simulink model "model"  (R2017b)
settings: Solver=VariableStepAuto  StartTime=0.0  StopTime=10.0  RelTol=1e-3  EnableMultiTasking=on
values from neighbouring files (symbols this model uses):
  A = zeros(5,5)    [kalmanfilter.m]    (also in model_2017.m = [[0  0   0   0                0             0   1           ; model_rough.m; model_v2.m = [[0  0   0   0                0             0   1           ; model_v3.m = [[0  0   0   0                0             0   1           )
  B = zeros(5,6)    [kalmanfilter.m]    (also in model_2017.m = [[0      0      0      0     ];                        [0   ; model_rough.m; model_v2.m = [[0      0      0      0     ];                        [0   ; model_v3.m = [[0      0      0      0      0      0             ];       )
  C = eye(5)    [kalmanfilter.m]    (also in model_2017.m = [[0  0   0   0   0   0   1   0   0   0   0   0]; model_rough.m; model_v2.m = [[0  0   0   0   0   0   1   0   0   0   0   0]; model_v3.m = [[0  0   0   0   0   0   1   0   0   0   0   0])
settings Model: Creator=nagamune  LastModifiedBy=Carter
settings DataIOCC: LimitDataPoints=on  SaveFormat=Array
settings OptimizationCC: LifeSpan=inf
settings DebuggingCC: SolverPrmCheckMsg=warning  SFUnexpectedBacktrackingDiag=warning  SFNoUnconditionalDefaultTransitionDiag=warning  SFExecutionAtInitializationDiag=none
settings HardwareCC: ProdBitPerPointer=32  ProdBitPerSizeT=32  ProdBitPerPtrDiffT=32  ProdLargestAtomicFloat=None  ProdIntDivRoundTo=Undefined  ProdEndianess=Unspecified  ProdWordSize=32  ProdHWDeviceType=32-bit Generic
settings ModelReferenceCC: PropagateSignalLabelsOutOfModel=off
settings CodeAppCC: StateflowObjectComments=on
settings GRTTargetCC: TargetLangStandard=C89/C90 (ANSI)  GeneratePreprocessorConditionals=Disable all
settings ConfigComp: CovMetricSettings=dw  CovHtmlReporting=on  CovSaveCumulativeToWorkspaceVar=on  CovSaveSingleToWorkspaceVar=on  CovExternalEMLEnable=off  CovSFcnEnable=off

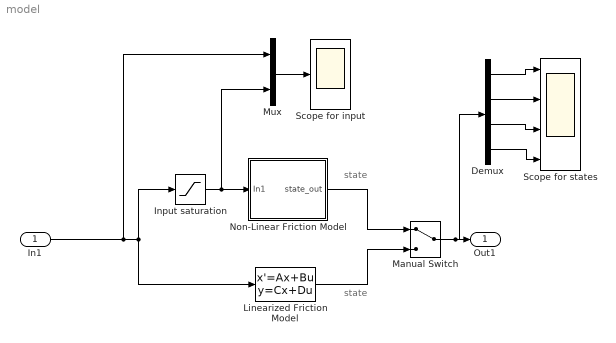
== system model ==
  note: state
  note: state
  In1 : Inport
  Demux : Demux
  Input saturation : Saturate  UpperLimit=10  LowerLimit=-10
  Linearized Friction Model : StateSpace  A=A  B=B  C=C  D=zeros(5,6)  InitialCondition=[0.3 0 0 0 0]
  Manual Switch : ManualSwitch
  Mux : Mux  Inputs=2
  Non-Linear Friction Model : Subsystem
  Scope for input : Scope
  Scope for states : Scope  NumInputPorts=4
  Out1 : Outport
  wires:
  Non-Linear Friction Model/1(state_out) -> Manual Switch/1
  Linearized Friction Model/1 -> Manual Switch/2
  In1/1 -> Mux/1, Linearized Friction Model/1, Input saturation/1
  Manual Switch/1 -> Demux/1, Out1/1
  Input saturation/1 -> Mux/2, Non-Linear Friction Model/1(In1)
  Demux/1 -> Scope for states/1
  Demux/2 -> Scope for states/2
  Demux/3 -> Scope for states/3
  Demux/4 -> Scope for states/4
  Mux/1 -> Scope for input/1

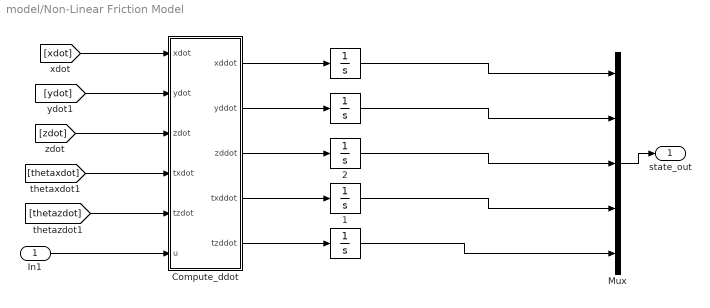
== system model/Non-Linear Friction Model ==
  In1 : Inport
  "  " : Integrator
  "   " : Integrator  InitialCondition=0.3
  "    " : Integrator
  "  1" : Integrator
  "  2" : Integrator
  Compute_ddot : MATLAB Function  TreatAsAtomicUnit=on
  Mux : Mux  Inputs=5
  state_out : Outport
  wires:
  In1/1 -> Compute_ddot/6(u)
  [thetaxdot] -> Compute_ddot/4(txdot)
  [zdot] -> Compute_ddot/3(zdot)
  [ydot] -> Compute_ddot/2(ydot)
  Compute_ddot/2(yddot) -> "    "/1
  [xdot] -> Compute_ddot/1(xdot)
  Mux/1 -> state_out/1
  [thetazdot] -> Compute_ddot/5(tzdot)
  Compute_ddot/5(tzddot) -> "  "/1
  Compute_ddot/1(xddot) -> "   "/1
  "   "/1 -> Mux/1
  "  "/1 -> Mux/5
  "  1"/1 -> Mux/4
  Compute_ddot/4(txddot) -> "  1"/1
  Compute_ddot/3(zddot) -> "  2"/1
  "  2"/1 -> Mux/3
  "    "/1 -> Mux/2

== matlab function model/Non-Linear Friction Model/Compute_ddot ==
  data: xddot output; xdot input; ydot input; yddot output; zdot input; txdot input; tzdot input; zddot output; txddot output; tzddot output; u input
function [xddot, yddot, zddot, txddot, tzddot] = get_ddot(xdot, ydot, zdot, txdot, tzdot, u)

% Load inertia, added inertia
m = 24.5;
ma_x = 12.8340;
ma_y = 17.3295;
ma_z = 21.9371;
I_x = 1.7047;
I_z = 1.6031;

% Load friction parameters and thruster matrix
% Friction = k_L*v + k_Q*v^2

% TEMP
k_Lx = 0.3;
k_Ly = 0.3;
k_Lz = 0.3;
k_Ltx = 0.3;
k_Ltz = 0.3;

k_Qx = 0.3;z
k_Qy = 0.3;
k_Qz = 0.3;
k_Qtx = 0.3;
k_Qtz = 0.3;

L_diags = 0.48; 
L_sides = 0.21;
B = zeros(5,6); 
B(1,:) = [cosd(45) cosd(45) cosd(45) cosd(45) 0 0];
B(2,:) = [cosd(45) -cosd(45) cosd(45) -cosd(45) 0 0];
B(3,:) = [ 0 0 0 0 1 1];
B(4,:) = [ 0 0 0 0 -L_sides L_sides];
B(5,:) = [-L_diags L_diags L_diags -L_diags 0 0];

% Standard for input u
% u = [F_sf, F_pf, F_sb, F_pb, F_st, F_pt]
% port, starboard, front, back, top
F_combo = B*u;

% Compute linear forces and torques F_x, F_y, F_z, T_x, T_z
xddot = (F_combo(1) - k_Lx*(xdot) -k_Qx*abs(xdot^2))/(m+ma_x);
yddot = (F_combo(2) - k_Ly*(ydot) -k_Qy*abs(ydot^2))/(m+ma_y);
zddot = (F_combo(3) - k_Lz*(zdot) -k_Qz*abs(zdot^2))/(m+ma_z);

txddot = (F_combo(4) - k_Ltx*(txdot) -k_Qtx*abs(txdot^2))/I_x;
tzddot = (F_combo(5) - k_Ltz*(tzdot) -k_Qtz*abs(tzdot^2))/I_z;
